simulink model "DARM"  (Simulink 7.5)
settings: Solver=ode45  StartTime=0.0  StopTime=10.0  RelTol=1e-3
values from neighbouring files (symbols this model uses):
  ifoParams = evalin('base', 'ifoParams')    [darmNbParams.m]
libraries: cstblocks x132, NbLibrary x29
(part 2 of 2)

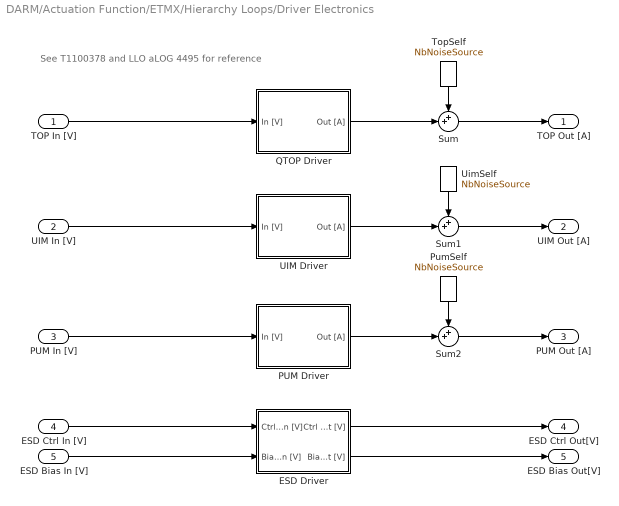
== system DARM/Actuation Function/ETMX/Hierarchy Loops/Driver Electronics ==
  note: See T1100378 and LLO aLOG 4495 for reference
  TOP In [V] : Inport
  UIM In [V] : Inport  Port=2
  PUM In [V] : Inport  Port=3
  ESD Ctrl In [V] : Inport  Port=4
  ESD Bias In [V] : Inport  Port=5
  ESD Driver : Subsystem
  PUM Driver : Subsystem  Description=FlexTf: ifoParams.act.drivers.pum.frd
      settings: AttributesFormatString=%<Description>
  PumSelf : NbLibrary/NbNoiseSource  Tag=NbNoiseSource  SystemSampleTime=-1  group='QUAD Actuator'  asd=ifoParams.darmNb.quadPumSelf
      settings: AttributesFormatString=%<Tag>
  QTOP Driver : Subsystem  Description=FlexTf: ifoParams.act.drivers.top.frd
      settings: AttributesFormatString=%<Description>
  Sum : Sum  Inputs=++|
  Sum1 : Sum  Inputs=++|
  Sum2 : Sum  Inputs=++|
  TopSelf : NbLibrary/NbNoiseSource  Tag=NbNoiseSource  SystemSampleTime=-1  group='QUAD Actuator'  asd=ifoParams.darmNb.quadTopSelf
      settings: AttributesFormatString=%<Tag>
  UIM Driver : Subsystem  Description=FlexTf: ifoParams.act.drivers.uim.frd
      settings: AttributesFormatString=%<Description>
  UimSelf : NbLibrary/NbNoiseSource  Tag=NbNoiseSource  SystemSampleTime=-1  group='QUAD Actuator'  asd=ifoParams.darmNb.quadUimSelf
      settings: AttributesFormatString=%<Tag>
  TOP Out [A] : Outport
  UIM Out [A] : Outport  Port=2
  PUM Out [A] : Outport  Port=3
  ESD Ctrl Out[V] : Outport  Port=4
  ESD Bias Out[V] : Outport  Port=5
  wires:
  TOP In [V]/1 -> QTOP Driver/1(In [V])
  PUM In [V]/1 -> PUM Driver/1(In [V])
  UIM In [V]/1 -> UIM Driver/1(In [V])
  ESD Driver/1(Ctrl Out [V]) -> ESD Ctrl Out[V]/1
  ESD Ctrl In [V]/1 -> ESD Driver/1(Ctrl In [V])
  ESD Driver/2(Bias Out [V]) -> ESD Bias Out[V]/1
  ESD Bias In [V]/1 -> ESD Driver/2(Bias In [V])
  TopSelf/1 -> Sum/1
  QTOP Driver/1(Out [A]) -> Sum/2
  Sum/1 -> TOP Out [A]/1
  UIM Driver/1(Out [A]) -> Sum1/2
  UimSelf/1 -> Sum1/1
  Sum1/1 -> UIM Out [A]/1
  PUM Driver/1(Out [A]) -> Sum2/2
  Sum2/1 -> PUM Out [A]/1
  PumSelf/1 -> Sum2/1

== system DARM/Actuation Function/ETMX/Hierarchy Loops/Driver Force Coefficient ==
  note: See T1100378
  note: Current to Force [N/A]
  note: Current to Force [N/A]
  note: Current to Force [N/A]
  In1[A] : Inport
  In2[A] : Inport  Port=2
  In3[A] : Inport  Port=3
  Vsig[V] : Inport  Port=4
  Vbias[V] : Inport  Port=5
  Gain : Gain  Gain=1.694
  Gain1 : Gain  Gain=1.694
  Gain2 : Gain  Gain=0.0309
  Gain7 : Gain  Gain=4.2e-10 / 4
  Math Function : Math  Operator=square  SaturateOnIntegerOverflow=on
  Subtract : Sum  Inputs=+-
  TOP_Out [N] : Outport
  UIM_Out [N] : Outport  Port=2
  PUM_Out [N] : Outport  Port=3
  TST_Out [N] : Outport  Port=4
  wires:
  In3[A]/1 -> Gain2/1
  In2[A]/1 -> Gain1/1
  In1[A]/1 -> Gain/1
  Gain2/1 -> PUM_Out [N]/1
  Gain1/1 -> UIM_Out [N]/1
  Gain/1 -> TOP_Out [N]/1
  Vsig[V]/1 -> Subtract/1
  Subtract/1 -> Math Function/1
  Math Function/1 -> Gain7/1
  Gain7/1 -> TST_Out [N]/1
  Vbias[V]/1 -> Subtract/2

== system DARM/Actuation Function/ETMX/Hierarchy Loops/EUL2OSEM ==
  note: 4 coil-magnet
      | actuators
  note: 4 coil-magnet
      | actuators
  note: 2 coil-magnet
      | actuators
  note: 4 ESD Quadrants
  M0_L_IN [ct] : Inport
  L1_L_IN [ct] : Inport  Port=2
  L2_L_IN [ct] : Inport  Port=3
  L3_L_IN [ct] : Inport  Port=4
  Gain1 : Gain  Gain=1/4
  Gain3 : Gain  Gain=1/2
  Gain4 : Gain  Gain=1/4
  Gain5 : Gain  Gain=1/4
  M0_OSEM_OUT [ct] : Outport
  L1_OSEM_OUT [ct] : Outport  Port=2
  L2_OSEM_OUT [ct] : Outport  Port=3
  L3_OSEM_OUT [ct] : Outport  Port=4
  wires:
  M0_L_IN [ct]/1 -> Gain3/1
  L1_L_IN [ct]/1 -> Gain4/1
  L2_L_IN [ct]/1 -> Gain5/1
  L3_L_IN [ct]/1 -> Gain1/1
  Gain3/1 -> M0_OSEM_OUT [ct]/1
  Gain4/1 -> L1_OSEM_OUT [ct]/1
  Gain5/1 -> L2_OSEM_OUT [ct]/1
  Gain1/1 -> L3_OSEM_OUT [ct]/1

== system DARM/Actuation Function/ETMX/Hierarchy Loops/L1 LOCK ==
  LSC_IN [m] : Inport
  FM1 : cstblocks/LTI System  Description=FlexTf: ifoParams.act.L1.lock(1).frd  SystemSampleTime=-1  sys=ifoParams.act.L1.lock(1).ss  IC=[]
      settings: AttributesFormatString=%<Description>
  FM10 : cstblocks/LTI System  SystemSampleTime=-1  sys=ifoParams.act.L1.lock(10).ss  IC=[]
  FM2 : cstblocks/LTI System  Description=FlexTf: ifoParams.act.L1.lock(2).frd  SystemSampleTime=-1  sys=ifoParams.act.L1.lock(2).ss  IC=[]
      settings: AttributesFormatString=%<Description>
  FM3 : cstblocks/LTI System  SystemSampleTime=-1  sys=ifoParams.act.L1.lock(3).ss  IC=[]
  FM4 : cstblocks/LTI System  SystemSampleTime=-1  sys=ifoParams.act.L1.lock(4).ss  IC=[]
  FM5 : cstblocks/LTI System  SystemSampleTime=-1  sys=ifoParams.act.L1.lock(5).ss  IC=[]
  FM6 : cstblocks/LTI System  SystemSampleTime=-1  sys=ifoParams.act.L1.lock(6).ss  IC=[]
  FM7 : cstblocks/LTI System  SystemSampleTime=-1  sys=ifoParams.act.L1.lock(7).ss  IC=[]
  FM8 : cstblocks/LTI System  SystemSampleTime=-1  sys=ifoParams.act.L1.lock(8).ss  IC=[]
  FM9 : cstblocks/LTI System  SystemSampleTime=-1  sys=ifoParams.act.L1.lock(9).ss  IC=[]
  Gain2 : Gain  Gain=ifoParams.act.L1.lockGain
  L1_OUT [ct] : Outport
  wires:
  FM1/1 -> FM2/1
  FM2/1 -> FM3/1
  FM3/1 -> FM4/1
  FM4/1 -> FM5/1
  FM6/1 -> FM7/1
  FM7/1 -> FM8/1
  FM8/1 -> FM9/1
  FM9/1 -> FM10/1
  LSC_IN [m]/1 -> FM1/1
  FM10/1 -> Gain2/1
  Gain2/1 -> L1_OUT [ct]/1
  FM5/1 -> FM6/1

== system DARM/Actuation Function/ETMX/Hierarchy Loops/L2 LOCK ==
  LSC_IN [m] : Inport
  FM1 : cstblocks/LTI System  Description=FlexTf: ifoParams.act.L2.lock(1).frd  SystemSampleTime=-1  sys=ifoParams.act.L2.lock(1).ss  IC=[]
      settings: AttributesFormatString=%<Description>
  FM10 : cstblocks/LTI System  SystemSampleTime=-1  sys=ifoParams.act.L2.lock(10).ss  IC=[]
  FM2 : cstblocks/LTI System  Description=FlexTf: ifoParams.act.L2.lock(2).frd  SystemSampleTime=-1  sys=ifoParams.act.L2.lock(2).ss  IC=[]
      settings: AttributesFormatString=%<Description>
  FM3 : cstblocks/LTI System  Description=FlexTf: ifoParams.act.L2.lock(3).frd  SystemSampleTime=-1  sys=ifoParams.act.L2.lock(3).ss  IC=[]
      settings: AttributesFormatString=%<Description>
  FM4 : cstblocks/LTI System  SystemSampleTime=-1  sys=ifoParams.act.L2.lock(4).ss  IC=[]
  FM5 : cstblocks/LTI System  SystemSampleTime=-1  sys=ifoParams.act.L2.lock(5).ss  IC=[]
  FM6 : cstblocks/LTI System  SystemSampleTime=-1  sys=ifoParams.act.L2.lock(6).ss  IC=[]
  FM7 : cstblocks/LTI System  SystemSampleTime=-1  sys=ifoParams.act.L2.lock(7).ss  IC=[]
  FM8 : cstblocks/LTI System  SystemSampleTime=-1  sys=ifoParams.act.L2.lock(8).ss  IC=[]
  FM9 : cstblocks/LTI System  SystemSampleTime=-1  sys=ifoParams.act.L2.lock(9).ss  IC=[]
  Gain2 : Gain  Gain=ifoParams.act.L2.lockGain
  L2_OUT [ct] : Outport
  wires:
  FM1/1 -> FM2/1
  FM2/1 -> FM3/1
  FM3/1 -> FM4/1
  FM4/1 -> FM5/1
  FM6/1 -> FM7/1
  FM7/1 -> FM8/1
  FM8/1 -> FM9/1
  FM9/1 -> FM10/1
  LSC_IN [m]/1 -> FM1/1
  FM10/1 -> Gain2/1
  Gain2/1 -> L2_OUT [ct]/1
  FM5/1 -> FM6/1

== system DARM/Actuation Function/ETMX/Hierarchy Loops/L3 LOCK ==
  LSC_IN [m] : Inport
  FM1 : cstblocks/LTI System  Description=FlexTf: ifoParams.act.L3.lock(1).frd  SystemSampleTime=-1  sys=ifoParams.act.L3.lock(1).ss  IC=[]
      settings: AttributesFormatString=%<Description>
  FM10 : cstblocks/LTI System  SystemSampleTime=-1  sys=ifoParams.act.L3.lock(10).ss  IC=[]
  FM2 : cstblocks/LTI System  Description=FlexTf: ifoParams.act.L3.lock(2).frd  SystemSampleTime=-1  sys=ifoParams.act.L3.lock(2).ss  IC=[]
      settings: AttributesFormatString=%<Description>
  FM3 : cstblocks/LTI System  Description=FlexTf: ifoParams.act.L3.lock(3).frd  SystemSampleTime=-1  sys=ifoParams.act.L3.lock(3).ss  IC=[]
      settings: AttributesFormatString=%<Description>
  FM4 : cstblocks/LTI System  SystemSampleTime=-1  sys=ifoParams.act.L3.lock(4).ss  IC=[]
  FM5 : cstblocks/LTI System  SystemSampleTime=-1  sys=ifoParams.act.L3.lock(5).ss  IC=[]
  FM6 : cstblocks/LTI System  SystemSampleTime=-1  sys=ifoParams.act.L3.lock(6).ss  IC=[]
  FM7 : cstblocks/LTI System  SystemSampleTime=-1  sys=ifoParams.act.L3.lock(7).ss  IC=[]
  FM8 : cstblocks/LTI System  SystemSampleTime=-1  sys=ifoParams.act.L3.lock(8).ss  IC=[]
  FM9 : cstblocks/LTI System  SystemSampleTime=-1  sys=ifoParams.act.L3.lock(9).ss  IC=[]
  Gain2 : Gain  Gain=ifoParams.act.L3.lockGain
  L3_OUT [ct] : Outport
  wires:
  FM1/1 -> FM2/1
  FM2/1 -> FM3/1
  FM3/1 -> FM4/1
  FM4/1 -> FM5/1
  FM6/1 -> FM7/1
  FM7/1 -> FM8/1
  FM8/1 -> FM9/1
  FM9/1 -> FM10/1
  LSC_IN [m]/1 -> FM1/1
  FM10/1 -> Gain2/1
  Gain2/1 -> L3_OUT [ct]/1
  FM5/1 -> FM6/1

== system DARM/Actuation Function/ETMX/Hierarchy Loops/LSC_ETMX ==
  LSC_ETMX_IN : Inport
  FM1 : cstblocks/LTI System  SystemSampleTime=-1  sys=ifoParams.act.lsc.etmx(1).ss  IC=[]
  FM10 : cstblocks/LTI System  SystemSampleTime=-1  sys=ifoParams.act.lsc.etmx(10).ss  IC=[]
  FM2 : cstblocks/LTI System  SystemSampleTime=-1  sys=ifoParams.act.lsc.etmx(2).ss  IC=[]
  FM3 : cstblocks/LTI System  SystemSampleTime=-1  sys=ifoParams.act.lsc.etmx(3).ss  IC=[]
  FM4 : cstblocks/LTI System  SystemSampleTime=-1  sys=ifoParams.act.lsc.etmx(4).ss  IC=[]
  FM5 : cstblocks/LTI System  SystemSampleTime=-1  sys=ifoParams.act.lsc.etmx(5).ss  IC=[]
  FM6 : cstblocks/LTI System  SystemSampleTime=-1  sys=ifoParams.act.lsc.etmx(6).ss  IC=[]
  FM7 : cstblocks/LTI System  SystemSampleTime=-1  sys=ifoParams.act.lsc.etmx(7).ss  IC=[]
  FM8 : cstblocks/LTI System  SystemSampleTime=-1  sys=ifoParams.act.lsc.etmx(8).ss  IC=[]
  FM9 : cstblocks/LTI System  SystemSampleTime=-1  sys=ifoParams.act.lsc.etmx(9).ss  IC=[]
  Gain2 : Gain  Gain=ifoParams.act.lsc.etmxGain
  "LSC_ETMX_OUT " : Outport
  wires:
  FM1/1 -> FM2/1
  FM2/1 -> FM3/1
  FM3/1 -> FM4/1
  FM4/1 -> FM5/1
  FM6/1 -> FM7/1
  FM7/1 -> FM8/1
  FM8/1 -> FM9/1
  FM9/1 -> FM10/1
  LSC_ETMX_IN/1 -> FM1/1
  FM10/1 -> Gain2/1
  Gain2/1 -> "LSC_ETMX_OUT "/1
  FM5/1 -> FM6/1

== system DARM/Actuation Function/ETMX/Hierarchy Loops/M0 LOCK ==
  LSC_IN [m] : Inport
  FM1 : cstblocks/LTI System  SystemSampleTime=-1  sys=ifoParams.act.M0.lock(1).ss  IC=[]
  FM10 : cstblocks/LTI System  SystemSampleTime=-1  sys=ifoParams.act.M0.lock(10).ss  IC=[]
  FM2 : cstblocks/LTI System  SystemSampleTime=-1  sys=ifoParams.act.M0.lock(2).ss  IC=[]
  FM3 : cstblocks/LTI System  SystemSampleTime=-1  sys=ifoParams.act.M0.lock(3).ss  IC=[]
  FM4 : cstblocks/LTI System  SystemSampleTime=-1  sys=ifoParams.act.M0.lock(4).ss  IC=[]
  FM5 : cstblocks/LTI System  SystemSampleTime=-1  sys=ifoParams.act.M0.lock(5).ss  IC=[]
  FM6 : cstblocks/LTI System  SystemSampleTime=-1  sys=ifoParams.act.M0.lock(6).ss  IC=[]
  FM7 : cstblocks/LTI System  SystemSampleTime=-1  sys=ifoParams.act.M0.lock(7).ss  IC=[]
  FM8 : cstblocks/LTI System  SystemSampleTime=-1  sys=ifoParams.act.M0.lock(8).ss  IC=[]
  FM9 : cstblocks/LTI System  SystemSampleTime=-1  sys=ifoParams.act.M0.lock(9).ss  IC=[]
  Gain2 : Gain  Gain=ifoParams.act.M0.lockGain
  M0_OUT [ct] : Outport
  wires:
  FM1/1 -> FM2/1
  FM2/1 -> FM3/1
  FM3/1 -> FM4/1
  FM4/1 -> FM5/1
  FM6/1 -> FM7/1
  FM7/1 -> FM8/1
  FM8/1 -> FM9/1
  FM9/1 -> FM10/1
  LSC_IN [m]/1 -> FM1/1
  FM10/1 -> Gain2/1
  Gain2/1 -> M0_OUT [ct]/1
  FM5/1 -> FM6/1

== system DARM/Actuation Function/ETMY/Hierarchy Loops/Actuator-to-Euler Transform ==
  note: 4 coil-magnet
      | actuators
  note: 4 coil-magnet
      | actuators
  note: 2 coil-magnet
      | actuators
  note: 4 ESD Quadrants
  TOP_OSEM_IN [N] : Inport
  UIM_OSEM_IN [N] : Inport  Port=2
  PUM_OSEM_IN [N] : Inport  Port=3
  TST_OSEM_IN [N] : Inport  Port=4
  Gain1 : Gain  Gain=4
  Gain3 : Gain  Gain=2
  Gain4 : Gain  Gain=4
  Gain5 : Gain  Gain=4
  TOP_L_OUT [N] : Outport
  UIM_L_OUT [N] : Outport  Port=2
  PUM_L_OUT [N] : Outport  Port=3
  TST_L_OUT [N] : Outport  Port=4
  wires:
  TOP_OSEM_IN [N]/1 -> Gain3/1
  Gain3/1 -> TOP_L_OUT [N]/1
  UIM_OSEM_IN [N]/1 -> Gain4/1
  Gain4/1 -> UIM_L_OUT [N]/1
  PUM_OSEM_IN [N]/1 -> Gain5/1
  Gain5/1 -> PUM_L_OUT [N]/1
  TST_OSEM_IN [N]/1 -> Gain1/1
  Gain1/1 -> TST_L_OUT [N]/1

== system DARM/Actuation Function/ETMY/Hierarchy Loops/Anti-Aliasing Chassis ==
  TOP In [V[ : Inport
  UIM In [V] : Inport  Port=2
  PUM In [V] : Inport  Port=3
  ESD Ctrl In [V] : Inport  Port=4
  ESD Bias In [V] : Inport  Port=5
  Gain{,1..4} (5 alike) : Gain
  TOP Out [V] : Outport
  UIM Out [V] : Outport  Port=2
  PUM Out[V] : Outport  Port=3
  ESD Ctrl Out V] : Outport  Port=4
  ESD Bias Out [V] : Outport  Port=5
  wires:
  Gain1/1 -> UIM Out [V]/1
  UIM In [V]/1 -> Gain1/1
  Gain2/1 -> PUM Out[V]/1
  PUM In [V]/1 -> Gain2/1
  Gain/1 -> TOP Out [V]/1
  TOP In [V[/1 -> Gain/1
  Gain3/1 -> ESD Ctrl Out V]/1
  ESD Ctrl In [V]/1 -> Gain3/1
  Gain4/1 -> ESD Bias Out [V]/1
  ESD Bias In [V]/1 -> Gain4/1

== system DARM/Actuation Function/ETMY/Hierarchy Loops/COILOUTF ==
  note: See T1100378 and LLO aLOG 4495 for reference
  M0_IN [ct] : Inport
  L1_IN [ct] : Inport  Port=2
  L2_IN [ct] : Inport  Port=3
  L3_CTRL_IN [ct] : Inport  Port=4
  L3_BIAS_IN [ct] : Inport  Port=5
  L1 : Subsystem
  L2 : Subsystem
  L3 : Subsystem
  M0 : Subsystem
  M0_OUT [ct] : Outport
  L1_OUT [ct] : Outport  Port=2
  L2_OUT [ct] : Outport  Port=3
  L3_CTRL_OUT [ct] : Outport  Port=4
  L3_BIAS_OUT [ct] : Outport  Port=5
  wires:
  M0/1(Out [ct]) -> M0_OUT [ct]/1
  M0_IN [ct]/1 -> M0/1(In [ct])
  L2_IN [ct]/1 -> L2/1(In [ct])
  L1_IN [ct]/1 -> L1/1(In [ct])
  L3/1(Ctrl Out [V]) -> L3_CTRL_OUT [ct]/1
  L3_CTRL_IN [ct]/1 -> L3/1(Ctrl In [V])
  L1/1(Out [ct]) -> L1_OUT [ct]/1
  L2/1(Out [ct]) -> L2_OUT [ct]/1
  L3/2(Bias Out [V]) -> L3_BIAS_OUT [ct]/1
  L3_BIAS_IN [ct]/1 -> L3/2(Bias In [V])

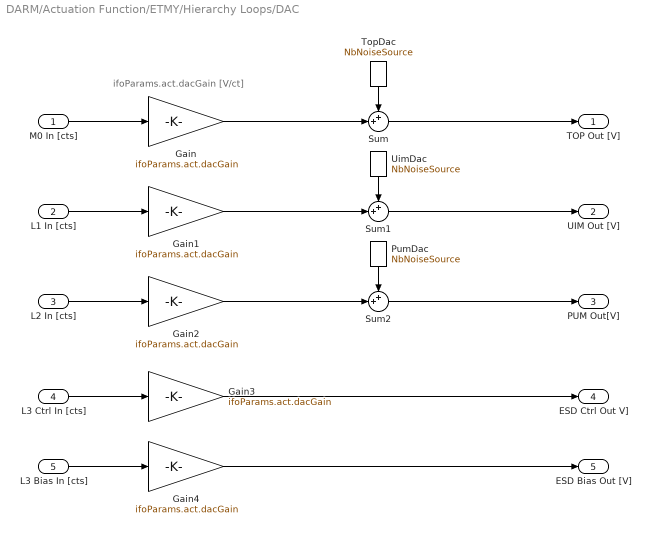
== system DARM/Actuation Function/ETMY/Hierarchy Loops/DAC ==
  note: ifoParams.act.dacGain
      | [V/ct]
  M0 In [cts] : Inport
  L1 In [cts] : Inport  Port=2
  L2 In [cts] : Inport  Port=3
  L3 Ctrl In [cts] : Inport  Port=4
  L3 Bias In [cts] : Inport  Port=5
  Gain{,1..4} (5 alike) : Gain  Gain=ifoParams.act.dacGain
  PumDac : NbLibrary/NbNoiseSource  Tag=NbNoiseSource  SystemSampleTime=-1  group='QUAD Actuator'  asd=ifoParams.darmNb.quadPumDac
      settings: AttributesFormatString=%<Tag>
  Sum : Sum  Inputs=++|
  Sum1 : Sum  Inputs=++|
  Sum2 : Sum  Inputs=++|
  TopDac : NbLibrary/NbNoiseSource  Tag=NbNoiseSource  SystemSampleTime=-1  group='QUAD Actuator'  asd=ifoParams.darmNb.quadTopDac
      settings: AttributesFormatString=%<Tag>
  UimDac : NbLibrary/NbNoiseSource  Tag=NbNoiseSource  SystemSampleTime=-1  group='QUAD Actuator'  asd=ifoParams.darmNb.quadUimDac
      settings: AttributesFormatString=%<Tag>
  TOP Out [V] : Outport
  UIM Out [V] : Outport  Port=2
  PUM Out[V] : Outport  Port=3
  ESD Ctrl Out V] : Outport  Port=4
  ESD Bias Out [V] : Outport  Port=5
  wires:
  L1 In [cts]/1 -> Gain1/1
  L2 In [cts]/1 -> Gain2/1
  M0 In [cts]/1 -> Gain/1
  L3 Ctrl In [cts]/1 -> Gain3/1
  Gain4/1 -> ESD Bias Out [V]/1
  L3 Bias In [cts]/1 -> Gain4/1
  Gain/1 -> Sum/2
  Sum/1 -> TOP Out [V]/1
  TopDac/1 -> Sum/1
  UimDac/1 -> Sum1/1
  Gain1/1 -> Sum1/2
  Sum1/1 -> UIM Out [V]/1
  Gain2/1 -> Sum2/2
  Sum2/1 -> PUM Out[V]/1
  PumDac/1 -> Sum2/1
  Gain3/1 -> ESD Ctrl Out V]/1

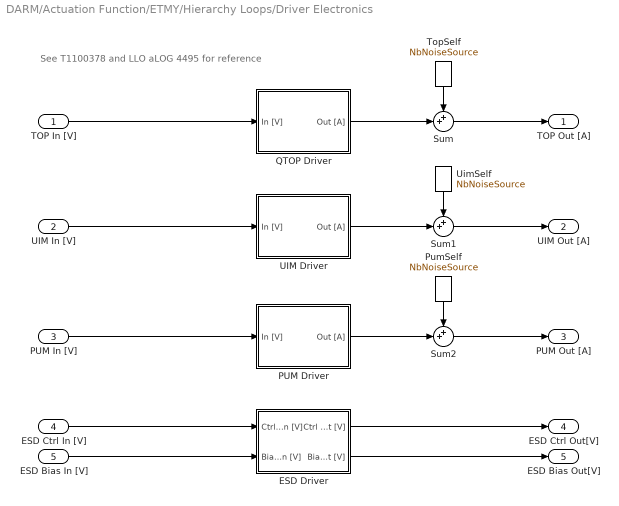
== system DARM/Actuation Function/ETMY/Hierarchy Loops/Driver Electronics ==
  note: See T1100378 and LLO aLOG 4495 for reference
  TOP In [V] : Inport
  UIM In [V] : Inport  Port=2
  PUM In [V] : Inport  Port=3
  ESD Ctrl In [V] : Inport  Port=4
  ESD Bias In [V] : Inport  Port=5
  ESD Driver : Subsystem
  PUM Driver : Subsystem  Description=FlexTf: ifoParams.act.drivers.pum.frd
      settings: AttributesFormatString=%<Description>
  PumSelf : NbLibrary/NbNoiseSource  Tag=NbNoiseSource  SystemSampleTime=-1  group='QUAD Actuator'  asd=ifoParams.darmNb.quadPumSelf
      settings: AttributesFormatString=%<Tag>
  QTOP Driver : Subsystem  Description=FlexTf: ifoParams.act.drivers.top.frd
      settings: AttributesFormatString=%<Description>
  Sum : Sum  Inputs=++|
  Sum1 : Sum  Inputs=++|
  Sum2 : Sum  Inputs=++|
  TopSelf : NbLibrary/NbNoiseSource  Tag=NbNoiseSource  SystemSampleTime=-1  group='QUAD Actuator'  asd=ifoParams.darmNb.quadTopSelf
      settings: AttributesFormatString=%<Tag>
  UIM Driver : Subsystem  Description=FlexTf: ifoParams.act.drivers.uim.frd
      settings: AttributesFormatString=%<Description>
  UimSelf : NbLibrary/NbNoiseSource  Tag=NbNoiseSource  SystemSampleTime=-1  group='QUAD Actuator'  asd=ifoParams.darmNb.quadUimSelf
      settings: AttributesFormatString=%<Tag>
  TOP Out [A] : Outport
  UIM Out [A] : Outport  Port=2
  PUM Out [A] : Outport  Port=3
  ESD Ctrl Out[V] : Outport  Port=4
  ESD Bias Out[V] : Outport  Port=5
  wires:
  TOP In [V]/1 -> QTOP Driver/1(In [V])
  PUM In [V]/1 -> PUM Driver/1(In [V])
  UIM In [V]/1 -> UIM Driver/1(In [V])
  ESD Driver/1(Ctrl Out [V]) -> ESD Ctrl Out[V]/1
  ESD Ctrl In [V]/1 -> ESD Driver/1(Ctrl In [V])
  ESD Driver/2(Bias Out [V]) -> ESD Bias Out[V]/1
  ESD Bias In [V]/1 -> ESD Driver/2(Bias In [V])
  QTOP Driver/1(Out [A]) -> Sum/2
  TopSelf/1 -> Sum/1
  Sum/1 -> TOP Out [A]/1
  UIM Driver/1(Out [A]) -> Sum1/2
  Sum1/1 -> UIM Out [A]/1
  UimSelf/1 -> Sum1/1
  PUM Driver/1(Out [A]) -> Sum2/2
  Sum2/1 -> PUM Out [A]/1
  PumSelf/1 -> Sum2/1

== system DARM/Actuation Function/ETMY/Hierarchy Loops/Driver Force Coefficient ==
  note: See T1100378
  note: Current to Force [N/A]
  note: Current to Force [N/A]
  note: Current to Force [N/A]
  In1[A] : Inport
  In2[A] : Inport  Port=2
  In3[A] : Inport  Port=3
  Vsig[V] : Inport  Port=4
  Vbias[V] : Inport  Port=5
  Gain : Gain  Gain=1.694
  Gain1 : Gain  Gain=1.694
  Gain2 : Gain  Gain=0.0309
  Gain7 : Gain  Gain=4.2e-10 / 4
  Math Function : Math  Operator=square  SaturateOnIntegerOverflow=on
  Subtract : Sum  Inputs=+-
  TOP_Out [N] : Outport
  UIM_Out [N] : Outport  Port=2
  PUM_Out [N] : Outport  Port=3
  TST_Out [N] : Outport  Port=4
  wires:
  In3[A]/1 -> Gain2/1
  In2[A]/1 -> Gain1/1
  In1[A]/1 -> Gain/1
  Gain2/1 -> PUM_Out [N]/1
  Gain1/1 -> UIM_Out [N]/1
  Gain/1 -> TOP_Out [N]/1
  Vsig[V]/1 -> Subtract/1
  Subtract/1 -> Math Function/1
  Math Function/1 -> Gain7/1
  Gain7/1 -> TST_Out [N]/1
  Vbias[V]/1 -> Subtract/2

== system DARM/Actuation Function/ETMY/Hierarchy Loops/EUL2OSEM ==
  note: 4 coil-magnet
      | actuators
  note: 4 coil-magnet
      | actuators
  note: 2 coil-magnet
      | actuators
  note: 4 ESD Quadrants
  M0_L_IN [ct] : Inport
  L1_L_IN [ct] : Inport  Port=2
  L2_L_IN [ct] : Inport  Port=3
  L3_L_IN [ct] : Inport  Port=4
  Gain1 : Gain  Gain=1/4
  Gain3 : Gain  Gain=1/2
  Gain4 : Gain  Gain=1/4
  Gain5 : Gain  Gain=1/4
  M0_OSEM_OUT [ct] : Outport
  L1_OSEM_OUT [ct] : Outport  Port=2
  L2_OSEM_OUT [ct] : Outport  Port=3
  L3_OSEM_OUT [ct] : Outport  Port=4
  wires:
  M0_L_IN [ct]/1 -> Gain3/1
  L1_L_IN [ct]/1 -> Gain4/1
  L2_L_IN [ct]/1 -> Gain5/1
  L3_L_IN [ct]/1 -> Gain1/1
  Gain3/1 -> M0_OSEM_OUT [ct]/1
  Gain4/1 -> L1_OSEM_OUT [ct]/1
  Gain5/1 -> L2_OSEM_OUT [ct]/1
  Gain1/1 -> L3_OSEM_OUT [ct]/1

== system DARM/Actuation Function/ETMY/Hierarchy Loops/L1 LOCK ==
  LSC_IN [m] : Inport
  FM1 : cstblocks/LTI System  Description=FlexTf: ifoParams.act.L1.lock(1).frd  SystemSampleTime=-1  sys=ifoParams.act.L1.lock(1).ss  IC=[]
      settings: AttributesFormatString=%<Description>
  FM10 : cstblocks/LTI System  SystemSampleTime=-1  sys=ifoParams.act.L1.lock(10).ss  IC=[]
  FM2 : cstblocks/LTI System  Description=FlexTf: ifoParams.act.L1.lock(2).frd  SystemSampleTime=-1  sys=ifoParams.act.L1.lock(2).ss  IC=[]
      settings: AttributesFormatString=%<Description>
  FM3 : cstblocks/LTI System  SystemSampleTime=-1  sys=ifoParams.act.L1.lock(3).ss  IC=[]
  FM4 : cstblocks/LTI System  SystemSampleTime=-1  sys=ifoParams.act.L1.lock(4).ss  IC=[]
  FM5 : cstblocks/LTI System  SystemSampleTime=-1  sys=ifoParams.act.L1.lock(5).ss  IC=[]
  FM6 : cstblocks/LTI System  SystemSampleTime=-1  sys=ifoParams.act.L1.lock(6).ss  IC=[]
  FM7 : cstblocks/LTI System  SystemSampleTime=-1  sys=ifoParams.act.L1.lock(7).ss  IC=[]
  FM8 : cstblocks/LTI System  SystemSampleTime=-1  sys=ifoParams.act.L1.lock(8).ss  IC=[]
  FM9 : cstblocks/LTI System  SystemSampleTime=-1  sys=ifoParams.act.L1.lock(9).ss  IC=[]
  Gain2 : Gain  Gain=ifoParams.act.L1.lockGain
  L1_OUT [ct] : Outport
  wires:
  FM1/1 -> FM2/1
  FM2/1 -> FM3/1
  FM3/1 -> FM4/1
  FM4/1 -> FM5/1
  FM6/1 -> FM7/1
  FM7/1 -> FM8/1
  FM8/1 -> FM9/1
  FM9/1 -> FM10/1
  LSC_IN [m]/1 -> FM1/1
  FM10/1 -> Gain2/1
  Gain2/1 -> L1_OUT [ct]/1
  FM5/1 -> FM6/1

== system DARM/Actuation Function/ETMY/Hierarchy Loops/L2 LOCK ==
  LSC_IN [m] : Inport
  FM1 : cstblocks/LTI System  Description=FlexTf: ifoParams.act.L2.lock(1).frd  SystemSampleTime=-1  sys=ifoParams.act.L2.lock(1).ss  IC=[]
      settings: AttributesFormatString=%<Description>
  FM10 : cstblocks/LTI System  SystemSampleTime=-1  sys=ifoParams.act.L2.lock(10).ss  IC=[]
  FM2 : cstblocks/LTI System  Description=FlexTf: ifoParams.act.L2.lock(2).frd  SystemSampleTime=-1  sys=ifoParams.act.L2.lock(2).ss  IC=[]
      settings: AttributesFormatString=%<Description>
  FM3 : cstblocks/LTI System  Description=FlexTf: ifoParams.act.L2.lock(3).frd  SystemSampleTime=-1  sys=ifoParams.act.L2.lock(3).ss  IC=[]
      settings: AttributesFormatString=%<Description>
  FM4 : cstblocks/LTI System  SystemSampleTime=-1  sys=ifoParams.act.L2.lock(4).ss  IC=[]
  FM5 : cstblocks/LTI System  SystemSampleTime=-1  sys=ifoParams.act.L2.lock(5).ss  IC=[]
  FM6 : cstblocks/LTI System  SystemSampleTime=-1  sys=ifoParams.act.L2.lock(6).ss  IC=[]
  FM7 : cstblocks/LTI System  SystemSampleTime=-1  sys=ifoParams.act.L2.lock(7).ss  IC=[]
  FM8 : cstblocks/LTI System  SystemSampleTime=-1  sys=ifoParams.act.L2.lock(8).ss  IC=[]
  FM9 : cstblocks/LTI System  SystemSampleTime=-1  sys=ifoParams.act.L2.lock(9).ss  IC=[]
  Gain2 : Gain  Gain=ifoParams.act.L2.lockGain
  L2_OUT [ct] : Outport
  wires:
  FM1/1 -> FM2/1
  FM2/1 -> FM3/1
  FM3/1 -> FM4/1
  FM4/1 -> FM5/1
  FM6/1 -> FM7/1
  FM7/1 -> FM8/1
  FM8/1 -> FM9/1
  FM9/1 -> FM10/1
  LSC_IN [m]/1 -> FM1/1
  FM10/1 -> Gain2/1
  Gain2/1 -> L2_OUT [ct]/1
  FM5/1 -> FM6/1

== system DARM/Actuation Function/ETMY/Hierarchy Loops/L3 LOCK ==
  LSC_IN [m] : Inport
  FM1 : cstblocks/LTI System  Description=FlexTf: ifoParams.act.L3.lock(1).frd  SystemSampleTime=-1  sys=ifoParams.act.L3.lock(1).ss  IC=[]
      settings: AttributesFormatString=%<Description>
  FM10 : cstblocks/LTI System  SystemSampleTime=-1  sys=ifoParams.act.L3.lock(10).ss  IC=[]
  FM2 : cstblocks/LTI System  Description=FlexTf: ifoParams.act.L3.lock(2).frd  SystemSampleTime=-1  sys=ifoParams.act.L3.lock(2).ss  IC=[]
      settings: AttributesFormatString=%<Description>
  FM3 : cstblocks/LTI System  Description=FlexTf: ifoParams.act.L3.lock(3).frd  SystemSampleTime=-1  sys=ifoParams.act.L3.lock(3).ss  IC=[]
      settings: AttributesFormatString=%<Description>
  FM4 : cstblocks/LTI System  SystemSampleTime=-1  sys=ifoParams.act.L3.lock(4).ss  IC=[]
  FM5 : cstblocks/LTI System  SystemSampleTime=-1  sys=ifoParams.act.L3.lock(5).ss  IC=[]
  FM6 : cstblocks/LTI System  SystemSampleTime=-1  sys=ifoParams.act.L3.lock(6).ss  IC=[]
  FM7 : cstblocks/LTI System  SystemSampleTime=-1  sys=ifoParams.act.L3.lock(7).ss  IC=[]
  FM8 : cstblocks/LTI System  SystemSampleTime=-1  sys=ifoParams.act.L3.lock(8).ss  IC=[]
  FM9 : cstblocks/LTI System  SystemSampleTime=-1  sys=ifoParams.act.L3.lock(9).ss  IC=[]
  Gain2 : Gain  Gain=ifoParams.act.L3.lockGain
  L3_OUT [ct] : Outport
  wires:
  FM1/1 -> FM2/1
  FM2/1 -> FM3/1
  FM3/1 -> FM4/1
  FM4/1 -> FM5/1
  FM6/1 -> FM7/1
  FM7/1 -> FM8/1
  FM8/1 -> FM9/1
  FM9/1 -> FM10/1
  LSC_IN [m]/1 -> FM1/1
  FM10/1 -> Gain2/1
  Gain2/1 -> L3_OUT [ct]/1
  FM5/1 -> FM6/1

== system DARM/Actuation Function/ETMY/Hierarchy Loops/LSC_ETMY ==
  LSC_ETMX_IN : Inport
  FM1 : cstblocks/LTI System  SystemSampleTime=-1  sys=ifoParams.act.lsc.etmx(1).ss  IC=[]
  FM10 : cstblocks/LTI System  SystemSampleTime=-1  sys=ifoParams.act.lsc.etmx(10).ss  IC=[]
  FM2 : cstblocks/LTI System  SystemSampleTime=-1  sys=ifoParams.act.lsc.etmx(2).ss  IC=[]
  FM3 : cstblocks/LTI System  SystemSampleTime=-1  sys=ifoParams.act.lsc.etmx(3).ss  IC=[]
  FM4 : cstblocks/LTI System  SystemSampleTime=-1  sys=ifoParams.act.lsc.etmx(4).ss  IC=[]
  FM5 : cstblocks/LTI System  SystemSampleTime=-1  sys=ifoParams.act.lsc.etmx(5).ss  IC=[]
  FM6 : cstblocks/LTI System  SystemSampleTime=-1  sys=ifoParams.act.lsc.etmx(6).ss  IC=[]
  FM7 : cstblocks/LTI System  SystemSampleTime=-1  sys=ifoParams.act.lsc.etmx(7).ss  IC=[]
  FM8 : cstblocks/LTI System  SystemSampleTime=-1  sys=ifoParams.act.lsc.etmx(8).ss  IC=[]
  FM9 : cstblocks/LTI System  SystemSampleTime=-1  sys=ifoParams.act.lsc.etmx(9).ss  IC=[]
  Gain2 : Gain  Gain=ifoParams.act.lsc.etmxGain
  "LSC_ETMX_OUT " : Outport
  wires:
  FM1/1 -> FM2/1
  FM2/1 -> FM3/1
  FM3/1 -> FM4/1
  FM4/1 -> FM5/1
  FM6/1 -> FM7/1
  FM7/1 -> FM8/1
  FM8/1 -> FM9/1
  FM9/1 -> FM10/1
  LSC_ETMX_IN/1 -> FM1/1
  FM10/1 -> Gain2/1
  Gain2/1 -> "LSC_ETMX_OUT "/1
  FM5/1 -> FM6/1

== system DARM/Actuation Function/ETMY/Hierarchy Loops/M0 LOCK ==
  LSC_IN [m] : Inport
  FM1 : cstblocks/LTI System  SystemSampleTime=-1  sys=ifoParams.act.M0.lock(1).ss  IC=[]
  FM10 : cstblocks/LTI System  SystemSampleTime=-1  sys=ifoParams.act.M0.lock(10).ss  IC=[]
  FM2 : cstblocks/LTI System  SystemSampleTime=-1  sys=ifoParams.act.M0.lock(2).ss  IC=[]
  FM3 : cstblocks/LTI System  SystemSampleTime=-1  sys=ifoParams.act.M0.lock(3).ss  IC=[]
  FM4 : cstblocks/LTI System  SystemSampleTime=-1  sys=ifoParams.act.M0.lock(4).ss  IC=[]
  FM5 : cstblocks/LTI System  SystemSampleTime=-1  sys=ifoParams.act.M0.lock(5).ss  IC=[]
  FM6 : cstblocks/LTI System  SystemSampleTime=-1  sys=ifoParams.act.M0.lock(6).ss  IC=[]
  FM7 : cstblocks/LTI System  SystemSampleTime=-1  sys=ifoParams.act.M0.lock(7).ss  IC=[]
  FM8 : cstblocks/LTI System  SystemSampleTime=-1  sys=ifoParams.act.M0.lock(8).ss  IC=[]
  FM9 : cstblocks/LTI System  SystemSampleTime=-1  sys=ifoParams.act.M0.lock(9).ss  IC=[]
  Gain2 : Gain  Gain=ifoParams.act.M0.lockGain
  M0_OUT [ct] : Outport
  wires:
  FM1/1 -> FM2/1
  FM2/1 -> FM3/1
  FM3/1 -> FM4/1
  FM4/1 -> FM5/1
  FM6/1 -> FM7/1
  FM7/1 -> FM8/1
  FM8/1 -> FM9/1
  FM9/1 -> FM10/1
  LSC_IN [m]/1 -> FM1/1
  FM10/1 -> Gain2/1
  Gain2/1 -> M0_OUT [ct]/1
  FM5/1 -> FM6/1

== system DARM/Sensing Function/DCPD Analog Electronics/Preamps/Preamp_PD1 ==
  note: Switches pass upper path if set to 1 (one),
      | lower path if set to 0 (zero)
  note: Zeros and Poles Derived from Schematic
      | (with more precision than the frequencies noted above the stages)
      | D060572-v1 (or B3).
  In [A] : Inport
  DC Transimpedance De-energized : Gain  Gain=100
  DC Transimpedance Energized : Gain  Gain=400
  Switch : Switch  Threshold=0.5
  Whitening_1  [7.3:79] : ZeroPole  Zeros=-2*pi*[7.3]  Poles=-2*pi*[79]  Gain=[79/7.3]
  Whitening_2 [7.3:79] : ZeroPole  Zeros=-2*pi*[7.3]  Poles=-2*pi*[79]  Gain=[79/7.3]
  ifoParams.sens.preamp.zswitch.state : Constant  Value=ifoParams.sens.preamp.zswitch.state
  Out [V] : Outport
  wires:
  In [A]/1 -> DC Transimpedance Energized/1, DC Transimpedance De-energized/1
  Whitening_2 [7.3:79]/1 -> Out [V]/1
  DC Transimpedance Energized/1 -> Switch/1
  Whitening_1  [7.3:79]/1 -> Whitening_2 [7.3:79]/1
  ifoParams.sens.preamp.zswitch.state/1 -> Switch/2
  DC Transimpedance De-energized/1 -> Switch/3
  Switch/1 -> Whitening_1  [7.3:79]/1

== system DARM/Sensing Function/DCPD Analog Electronics/Preamps/Preamp_PD2 ==
  note: Switches pass upper path if set to 1 (one),
      | lower path if set to 0 (zero)
  note: Zeros and Poles Derived from Schematic
      | (with more precision than the frequencies noted above the stages)
      | D060572-v1 (or B3).
  In [A] : Inport
  DC Transimpedance De-energized : Gain  Gain=100
  DC Transimpedance Energized : Gain  Gain=400
  Switch : Switch  Threshold=0.5
  Whitening_1  [7.3:79] : ZeroPole  Zeros=-2*pi*[7.3]  Poles=-2*pi*[79]  Gain=[79/7.3]
  Whitening_2 [7.3:79] : ZeroPole  Zeros=-2*pi*[7.3]  Poles=-2*pi*[79]  Gain=[79/7.3]
  ifoParams.sens.preamp.zswitch.state : Constant  Value=ifoParams.sens.preamp.zswitch.state
  Out [V] : Outport
  wires:
  In [A]/1 -> DC Transimpedance Energized/1, DC Transimpedance De-energized/1
  Whitening_2 [7.3:79]/1 -> Out [V]/1
  DC Transimpedance Energized/1 -> Switch/1
  Whitening_1  [7.3:79]/1 -> Whitening_2 [7.3:79]/1
  ifoParams.sens.preamp.zswitch.state/1 -> Switch/2
  DC Transimpedance De-energized/1 -> Switch/3
  Switch/1 -> Whitening_1  [7.3:79]/1

== system DARM/Sensing Function/DCPD Analog Electronics/Whitening Chassis/Whitening_PD1 ==
  note: Switches pass upper path if set to 1 (one),
      | lower path if set to 0 (zero)
  note: Zeros and Poles Derived from Schematic
      | (with more precision than the frequencies noted above the stages)
      | D070281-v1
  In [V] : Inport
  DC Gain : Gain  Gain=0.5
  Switch : Switch  Threshold=0.5
  Switch1 : Switch  Threshold=0.5
  Whitening_1  [7.3:79] : ZeroPole  Zeros=-2*pi*[7.3]  Poles=-2*pi*[79]  Gain=[79/7.3]
  Whitening_2 [24:260] : ZeroPole  Zeros=-2*pi*[24]  Poles=-2*pi*[260]  Gain=[260/24]
  ifoParams.sens.whitening.stage1.state : Constant  Value=ifoParams.sens.whitening.stage1.state
  ifoParams.sens.whitening.stage2.state : Constant  Value=ifoParams.sens.whitening.stage2.state
  Out [V] : Outport
  wires:
  DC Gain/1 -> Switch/1, Whitening_1  [7.3:79]/1
  In [V]/1 -> DC Gain/1
  ifoParams.sens.whitening.stage1.state/1 -> Switch/2
  Whitening_1  [7.3:79]/1 -> Switch/3
  Whitening_2 [24:260]/1 -> Switch1/3
  Switch/1 -> Switch1/1, Whitening_2 [24:260]/1
  Switch1/1 -> Out [V]/1
  ifoParams.sens.whitening.stage2.state/1 -> Switch1/2

== system DARM/Sensing Function/DCPD Analog Electronics/Whitening Chassis/Whitening_PD2 ==
  note: Switches pass upper path if set to 1 (one),
      | lower path if set to 0 (zero)
  note: Zeros and Poles Derived from Schematic
      | (with more precision than the frequencies noted above the stages)
      | D070281-v1
  In [V] : Inport
  DC Gain : Gain  Gain=0.5
  Switch : Switch  Threshold=0.5
  Switch1 : Switch  Threshold=0.5
  Whitening_1  [7.3:79] : ZeroPole  Zeros=-2*pi*[7.3]  Poles=-2*pi*[79]  Gain=[79/7.3]
  Whitening_2 [24:260] : ZeroPole  Zeros=-2*pi*[24]  Poles=-2*pi*[260]  Gain=[260/24]
  ifoParams.sens.whitening.stage1.state : Constant  Value=ifoParams.sens.whitening.stage1.state
  ifoParams.sens.whitening.stage2.state : Constant  Value=ifoParams.sens.whitening.stage2.state
  Out [V] : Outport
  wires:
  DC Gain/1 -> Switch/1, Whitening_1  [7.3:79]/1
  In [V]/1 -> DC Gain/1
  ifoParams.sens.whitening.stage1.state/1 -> Switch/2
  Whitening_1  [7.3:79]/1 -> Switch/3
  Whitening_2 [24:260]/1 -> Switch1/3
  Switch/1 -> Switch1/1, Whitening_2 [24:260]/1
  Switch1/1 -> Out [V]/1
  ifoParams.sens.whitening.stage2.state/1 -> Switch1/2

== system DARM/Sensing Function/DCPD Signal Conditioning/ISCINF/AntiPreamps_PD1 ==
  In [ct] : Inport
  AntiWhitening_1  [7.3:79] : ZeroPole  Zeros=-2*pi*[79]  Poles=-2*pi*[7.3]  Gain=[7.3/79]
  AntiWhitening_2  [7.3:79] : ZeroPole  Zeros=-2*pi*[79]  Poles=-2*pi*[7.3]  Gain=[7.3/79]
  Out [ct] : Outport
  wires:
  AntiWhitening_1  [7.3:79]/1 -> AntiWhitening_2  [7.3:79]/1
  In [ct]/1 -> AntiWhitening_1  [7.3:79]/1
  AntiWhitening_2  [7.3:79]/1 -> Out [ct]/1

== system DARM/Sensing Function/DCPD Signal Conditioning/ISCINF/AntiPreamps_PD2 ==
  In [ct] : Inport
  AntiWhitening_1  [7.3:79] : ZeroPole  Zeros=-2*pi*[79]  Poles=-2*pi*[7.3]  Gain=[7.3/79]
  AntiWhitening_2  [7.3:79] : ZeroPole  Zeros=-2*pi*[79]  Poles=-2*pi*[7.3]  Gain=[7.3/79]
  Out [ct] : Outport
  wires:
  AntiWhitening_1  [7.3:79]/1 -> AntiWhitening_2  [7.3:79]/1
  In [ct]/1 -> AntiWhitening_1  [7.3:79]/1
  AntiWhitening_2  [7.3:79]/1 -> Out [ct]/1

== system DARM/Sensing Function/DCPD Signal Conditioning/ISCINF/AntiWhitening_PD1 ==
  note: Switches pass upper path if set to 1 (one),
      | lower path if set to 0 (zero)
  note: Zeros and Poles Derived from Schematic
      | (with more precision than the frequencies noted above the stages)
      | D070281-v1
  In [ct] : Inport
  AntiWhitening_1  [7.3:79] : ZeroPole  Zeros=-2*pi*[79]  Poles=-2*pi*[7.3]  Gain=[7.3/79]
  AntiWhitening_2 [24:260] : ZeroPole  Zeros=-2*pi*[260]  Poles=-2*pi*[24]  Gain=[24/260]
  Switch : Switch  Threshold=0.5
  Switch1 : Switch  Threshold=0.5
  ifoParams.sens.whitening.stage1.state : Constant  Value=ifoParams.sens.whitening.stage1.state
  ifoParams.sens.whitening.stage2.state : Constant  Value=ifoParams.sens.whitening.stage2.state
  Out [ct] : Outport
  wires:
  In [ct]/1 -> Switch/1, AntiWhitening_1  [7.3:79]/1
  ifoParams.sens.whitening.stage1.state/1 -> Switch/2
  AntiWhitening_1  [7.3:79]/1 -> Switch/3
  AntiWhitening_2 [24:260]/1 -> Switch1/3
  Switch/1 -> Switch1/1, AntiWhitening_2 [24:260]/1
  Switch1/1 -> Out [ct]/1
  ifoParams.sens.whitening.stage2.state/1 -> Switch1/2

== system DARM/Sensing Function/DCPD Signal Conditioning/ISCINF/AntiWhitening_PD2 ==
  note: Switches pass upper path if set to 1 (one),
      | lower path if set to 0 (zero)
  note: Zeros and Poles Derived from Schematic
      | (with more precision than the frequencies noted above the stages)
      | D070281-v1
  In [ct] : Inport
  AntiWhitening_1  [7.3:79] : ZeroPole  Zeros=-2*pi*[79]  Poles=-2*pi*[7.3]  Gain=[7.3/79]
  AntiWhitening_2 [24:260] : ZeroPole  Zeros=-2*pi*[260]  Poles=-2*pi*[24]  Gain=[24/260]
  Switch : Switch  Threshold=0.5
  Switch1 : Switch  Threshold=0.5
  ifoParams.sens.whitening.stage1.state : Constant  Value=ifoParams.sens.whitening.stage1.state
  ifoParams.sens.whitening.stage2.state : Constant  Value=ifoParams.sens.whitening.stage2.state
  Out [ct] : Outport
  wires:
  In [ct]/1 -> Switch/1, AntiWhitening_1  [7.3:79]/1
  ifoParams.sens.whitening.stage1.state/1 -> Switch/2
  AntiWhitening_1  [7.3:79]/1 -> Switch/3
  AntiWhitening_2 [24:260]/1 -> Switch1/3
  Switch/1 -> Switch1/1, AntiWhitening_2 [24:260]/1
  Switch1/1 -> Out [ct]/1
  ifoParams.sens.whitening.stage2.state/1 -> Switch1/2

== system DARM/Actuation Function/ETMX/Hierarchy Loops/COILOUTF/L1 ==
  note: Switches pass upper path if set to 1 (one),
      | lower path if set to 0 (zero)
  In [ct] : Inport
  Switch : Switch  Threshold=0.5
  Switch1 : Switch  Threshold=0.5
  Switch2 : Switch  Threshold=0.5
  antiAcq [10:1] : ZeroPole  Zeros=-2*pi*[300]  Poles=-2*pi*[50]  Gain=[50/300]
  antiLP1 [1:10.5] : ZeroPole  Zeros=-2*pi*[1]  Poles=-2*pi*[10.5]  Gain=[10.5/1]
  antiLP2 [1:10.5] : ZeroPole  Zeros=-2*pi*[1]  Poles=-2*pi*[10.5]  Gain=[10.5/1]
  antiLP3 [1:10.5] : ZeroPole  Zeros=-2*pi*[1]  Poles=-2*pi*[10.5]  Gain=[10.5/1]
  drivers.uim.state.lp1 : Constant  Value=ifoParams.act.drivers.uim.state.lp1
  drivers.uim.state.lp2 : Constant  Value=ifoParams.act.drivers.uim.state.lp2
  drivers.uim.state.lp3 : Constant  Value=ifoParams.act.drivers.uim.state.lp3
  Out [ct] : Outport
  wires:
  drivers.uim.state.lp1/1 -> Switch/2
  antiLP1 [1:10.5]/1 -> Switch/1
  Switch/1 -> Switch1/3, antiLP2 [1:10.5]/1
  antiLP2 [1:10.5]/1 -> Switch1/1
  drivers.uim.state.lp2/1 -> Switch1/2
  Switch1/1 -> Switch2/3, antiLP3 [1:10.5]/1
  antiLP3 [1:10.5]/1 -> Switch2/1
  drivers.uim.state.lp3/1 -> Switch2/2
  In [ct]/1 -> antiLP1 [1:10.5]/1, Switch/3
  Switch2/1 -> antiAcq [10:1]/1
  antiAcq [10:1]/1 -> Out [ct]/1

== system DARM/Actuation Function/ETMX/Hierarchy Loops/COILOUTF/L2 ==
  note: Switches pass upper path if set to 1 (one),
      | lower path if set to 0 (zero)
  In [ct] : Inport
  Switch : Switch  Threshold=0.5
  Switch1 : Switch  Threshold=0.5
  antiAcqOff [110:12] : ZeroPole  Zeros=-2*pi*[110]  Poles=-2*pi*[12]  Gain=12/110
  antiAcqOn [80.5:1.35] : ZeroPole  Zeros=-2*pi*[80.5]  Poles=-2*pi*[1.35]  Gain=1.35/80.5
  antiLpOn [(0.5 250):(6 20)] : ZeroPole  Zeros=-2*pi*[0.5 250]  Poles=-2*pi*[6 20]  Gain=(6*20)/(0.5*250)
  drivers.pum.state.lp : Constant  Value=ifoParams.act.drivers.pum.state.lp
  drivers.top.state.acq : Constant  Value=ifoParams.act.drivers.pum.state.acq
  Out [ct] : Outport
  wires:
  drivers.pum.state.lp/1 -> Switch/2
  Switch/1 -> antiAcqOn [80.5:1.35]/1, antiAcqOff [110:12]/1
  antiAcqOn [80.5:1.35]/1 -> Switch1/1
  drivers.top.state.acq/1 -> Switch1/2
  In [ct]/1 -> antiLpOn [(0.5 250):(6 20)]/1, Switch/3
  Switch1/1 -> Out [ct]/1
  antiLpOn [(0.5 250):(6 20)]/1 -> Switch/1
  antiAcqOff [110:12]/1 -> Switch1/3

== system DARM/Actuation Function/ETMX/Hierarchy Loops/COILOUTF/L3 ==
  note: 2 kHz Pole is not digitally compensated
  Ctrl In [V] : Inport
  Bias In [V] : Inport  Port=2
  Ctrl Out [V] : Outport
  Bias Out [V] : Outport  Port=2
  wires:
  Ctrl In [V]/1 -> Ctrl Out [V]/1
  Bias In [V]/1 -> Bias Out [V]/1

== system DARM/Actuation Function/ETMX/Hierarchy Loops/COILOUTF/M0 ==
  note: Switches pass upper path if set to 1 (one),
      | lower path if set to 0 (zero)
  In [ct] : Inport
  Switch : Switch  Threshold=0.5
  antiAcq [1:31] : ZeroPole  Zeros=-2*pi*[1]  Poles=-2*pi*[31]  Gain=[31/1]
  antiLP [1:10] : ZeroPole  Zeros=-2*pi*[1]  Poles=-2*pi*[10]  Gain=[10/1]
  drivers.top.state.lp : Constant  Value=ifoParams.act.drivers.top.state.lp
  Out [ct] : Outport
  wires:
  Switch/1 -> antiAcq [1:31]/1
  antiLP [1:10]/1 -> Switch/1
  In [ct]/1 -> antiLP [1:10]/1, Switch/3
  antiAcq [1:31]/1 -> Out [ct]/1
  drivers.top.state.lp/1 -> Switch/2

== system DARM/Actuation Function/ETMX/Hierarchy Loops/Driver Electronics/ESD Driver ==
  Ctrl In [V] : Inport
  Bias In [V] : Inport  Port=2
  DC Gain1 : Gain  Gain=1.1
  DC Gain3 : Gain  Gain=1.1
  L3_ESD_filter [(none):(2000)] : ZeroPole  Zeros=[]  Poles=-2*pi*[2000]  Gain=[2*pi*2000]
  L3_ESD_filter [(none):(2000)]1 : ZeroPole  Zeros=[]  Poles=-2*pi*[2000]  Gain=[2*pi*2000]
  Ctrl Out [V] : Outport
  Bias Out [V] : Outport  Port=2
  wires:
  DC Gain3/1 -> L3_ESD_filter [(none):(2000)]/1
  Ctrl In [V]/1 -> DC Gain3/1
  L3_ESD_filter [(none):(2000)]/1 -> Ctrl Out [V]/1
  Bias In [V]/1 -> DC Gain1/1
  DC Gain1/1 -> L3_ESD_filter [(none):(2000)]1/1
  L3_ESD_filter [(none):(2000)]1/1 -> Bias Out [V]/1

== system DARM/Actuation Function/ETMX/Hierarchy Loops/Driver Electronics/PUM Driver ==
  note: Switches pass upper path if set to 1 (one),
      | lower path if set to 0 (zero)
  In [V] : Inport
  DC Transconductance : Gain  Gain=0.27e-3
  L2_ACQOFF_filter [12:110] : ZeroPole  Zeros=-2*pi*[12]  Poles=-2*pi*[110]  Gain=110/12
  L2_ACQON_filter [1.35:80.5] : ZeroPole  Zeros=-2*pi*[1.35]  Poles=-2*pi*[80.5]  Gain=80.5/1.35
  L2_LPON_filter [(0.5 250):(6 20)] : ZeroPole  Zeros=-2*pi*[6 20]  Poles=-2*pi*[0.5 250]  Gain=(0.5*250)/(6*20)
  Switch : Switch  Threshold=0.5
  Switch1 : Switch  Threshold=0.5
  drivers.pum.state.lp : Constant  Value=ifoParams.act.drivers.pum.state.lp
  drivers.top.state.acq : Constant  Value=ifoParams.act.drivers.pum.state.acq
  Out [A] : Outport
  wires:
  DC Transconductance/1 -> L2_LPON_filter [(0.5 250):(6 20)]/1, Switch/3
  drivers.pum.state.lp/1 -> Switch/2
  Switch/1 -> L2_ACQOFF_filter [12:110]/1, L2_ACQON_filter [1.35:80.5]/1
  L2_ACQON_filter [1.35:80.5]/1 -> Switch1/1
  drivers.top.state.acq/1 -> Switch1/2
  In [V]/1 -> DC Transconductance/1
  Switch1/1 -> Out [A]/1
  L2_LPON_filter [(0.5 250):(6 20)]/1 -> Switch/1
  L2_ACQOFF_filter [12:110]/1 -> Switch1/3

== system DARM/Actuation Function/ETMX/Hierarchy Loops/Driver Electronics/QTOP Driver ==
  note: Switches pass upper path if set to 1 (one),
      | lower path if set to 0 (zero)
  In [V] : Inport
  DC Transconductance : Gain  Gain=9.9e-3
  LP_filter [10:1] : ZeroPole  Zeros=-2*pi*[10]  Poles=-2*pi*[1]  Gain=[1/10]
  M0_Output_Filter [31:0.9] : ZeroPole  Zeros=-2*pi*[31]  Poles=-2*pi*[0.9]  Gain=[0.9/31]
  Switch : Switch  Threshold=0.5
  drivers.top.state.lp : Constant  Value=ifoParams.act.drivers.top.state.lp
  Out [A] : Outport
  wires:
  Switch/1 -> M0_Output_Filter [31:0.9]/1
  LP_filter [10:1]/1 -> Switch/1
  DC Transconductance/1 -> LP_filter [10:1]/1, Switch/3
  In [V]/1 -> DC Transconductance/1
  M0_Output_Filter [31:0.9]/1 -> Out [A]/1
  drivers.top.state.lp/1 -> Switch/2

== system DARM/Actuation Function/ETMX/Hierarchy Loops/Driver Electronics/UIM Driver ==
  note: Switches pass upper path if set to 1 (one),
      | lower path if set to 0 (zero)
  In [V] : Inport
  DC Transconductance : Gain  Gain=0.15e-3
  L1_LP1_filter [10.5:1] : ZeroPole  Zeros=-2*pi*[10.5]  Poles=-2*pi*[1]  Gain=[1/10.5]
  L1_LP2_filter [10.5:1] : ZeroPole  Zeros=-2*pi*[10.5]  Poles=-2*pi*[1]  Gain=[1/10.5]
  L1_LP3_filter [10.5:1] : ZeroPole  Zeros=-2*pi*[10.5]  Poles=-2*pi*[1]  Gain=[1/10.5]
  L1_Output_filter [50:300] : ZeroPole  Zeros=-2*pi*[50]  Poles=-2*pi*[300]  Gain=[300/50]
  Switch : Switch  Threshold=0.5
  Switch1 : Switch  Threshold=0.5
  Switch2 : Switch  Threshold=0.5
  drivers.uim.state.lp1 : Constant  Value=ifoParams.act.drivers.uim.state.lp1
  drivers.uim.state.lp2 : Constant  Value=ifoParams.act.drivers.uim.state.lp2
  drivers.uim.state.lp3 : Constant  Value=ifoParams.act.drivers.uim.state.lp3
  Out [A] : Outport
  wires:
  DC Transconductance/1 -> L1_LP1_filter [10.5:1]/1, Switch/3
  drivers.uim.state.lp1/1 -> Switch/2
  L1_LP1_filter [10.5:1]/1 -> Switch/1
  Switch/1 -> L1_LP2_filter [10.5:1]/1, Switch1/3
  L1_LP2_filter [10.5:1]/1 -> Switch1/1
  drivers.uim.state.lp2/1 -> Switch1/2
  Switch1/1 -> L1_LP3_filter [10.5:1]/1, Switch2/3
  L1_LP3_filter [10.5:1]/1 -> Switch2/1
  drivers.uim.state.lp3/1 -> Switch2/2
  In [V]/1 -> DC Transconductance/1
  Switch2/1 -> L1_Output_filter [50:300]/1
  L1_Output_filter [50:300]/1 -> Out [A]/1

== system DARM/Actuation Function/ETMY/Hierarchy Loops/COILOUTF/L1 ==
  note: Switches pass upper path if set to 1 (one),
      | lower path if set to 0 (zero)
  In [ct] : Inport
  Switch : Switch  Threshold=0.5
  Switch1 : Switch  Threshold=0.5
  Switch2 : Switch  Threshold=0.5
  antiAcq [10:1] : ZeroPole  Zeros=-2*pi*[300]  Poles=-2*pi*[50]  Gain=[50/300]
  antiLP1 [1:10.5] : ZeroPole  Zeros=-2*pi*[1]  Poles=-2*pi*[10.5]  Gain=[10.5/1]
  antiLP2 [1:10.5] : ZeroPole  Zeros=-2*pi*[1]  Poles=-2*pi*[10.5]  Gain=[10.5/1]
  antiLP3 [1:10.5] : ZeroPole  Zeros=-2*pi*[1]  Poles=-2*pi*[10.5]  Gain=[10.5/1]
  drivers.uim.state.lp1 : Constant  Value=ifoParams.act.drivers.uim.state.lp1
  drivers.uim.state.lp2 : Constant  Value=ifoParams.act.drivers.uim.state.lp2
  drivers.uim.state.lp3 : Constant  Value=ifoParams.act.drivers.uim.state.lp3
  Out [ct] : Outport
  wires:
  drivers.uim.state.lp1/1 -> Switch/2
  antiLP1 [1:10.5]/1 -> Switch/1
  Switch/1 -> Switch1/3, antiLP2 [1:10.5]/1
  antiLP2 [1:10.5]/1 -> Switch1/1
  drivers.uim.state.lp2/1 -> Switch1/2
  Switch1/1 -> Switch2/3, antiLP3 [1:10.5]/1
  antiLP3 [1:10.5]/1 -> Switch2/1
  drivers.uim.state.lp3/1 -> Switch2/2
  In [ct]/1 -> antiLP1 [1:10.5]/1, Switch/3
  Switch2/1 -> antiAcq [10:1]/1
  antiAcq [10:1]/1 -> Out [ct]/1

== system DARM/Actuation Function/ETMY/Hierarchy Loops/COILOUTF/L2 ==
  note: Switches pass upper path if set to 1 (one),
      | lower path if set to 0 (zero)
  In [ct] : Inport
  Switch : Switch  Threshold=0.5
  Switch1 : Switch  Threshold=0.5
  antiAcqOff [110:12] : ZeroPole  Zeros=-2*pi*[110]  Poles=-2*pi*[12]  Gain=12/110
  antiAcqOn [80.5:1.35] : ZeroPole  Zeros=-2*pi*[80.5]  Poles=-2*pi*[1.35]  Gain=1.35/80.5
  antiLpOn [(0.5 250):(6 20)] : ZeroPole  Zeros=-2*pi*[0.5 250]  Poles=-2*pi*[6 20]  Gain=(6*20)/(0.5*250)
  drivers.pum.state.lp : Constant  Value=ifoParams.act.drivers.pum.state.lp
  drivers.top.state.acq : Constant  Value=ifoParams.act.drivers.pum.state.acq
  Out [ct] : Outport
  wires:
  drivers.pum.state.lp/1 -> Switch/2
  Switch/1 -> antiAcqOn [80.5:1.35]/1, antiAcqOff [110:12]/1
  antiAcqOn [80.5:1.35]/1 -> Switch1/1
  drivers.top.state.acq/1 -> Switch1/2
  In [ct]/1 -> antiLpOn [(0.5 250):(6 20)]/1, Switch/3
  Switch1/1 -> Out [ct]/1
  antiLpOn [(0.5 250):(6 20)]/1 -> Switch/1
  antiAcqOff [110:12]/1 -> Switch1/3

== system DARM/Actuation Function/ETMY/Hierarchy Loops/COILOUTF/L3 ==
  note: 2 kHz Pole is not digitally compensated
  Ctrl In [V] : Inport
  Bias In [V] : Inport  Port=2
  Ctrl Out [V] : Outport
  Bias Out [V] : Outport  Port=2
  wires:
  Ctrl In [V]/1 -> Ctrl Out [V]/1
  Bias In [V]/1 -> Bias Out [V]/1

== system DARM/Actuation Function/ETMY/Hierarchy Loops/COILOUTF/M0 ==
  note: Switches pass upper path if set to 1 (one),
      | lower path if set to 0 (zero)
  In [ct] : Inport
  Switch : Switch  Threshold=0.5
  antiAcq [1:31] : ZeroPole  Zeros=-2*pi*[1]  Poles=-2*pi*[31]  Gain=[31/1]
  antiLP [1:10] : ZeroPole  Zeros=-2*pi*[1]  Poles=-2*pi*[10]  Gain=[10/1]
  drivers.top.state.lp : Constant  Value=ifoParams.act.drivers.top.state.lp
  Out [ct] : Outport
  wires:
  Switch/1 -> antiAcq [1:31]/1
  antiLP [1:10]/1 -> Switch/1
  In [ct]/1 -> antiLP [1:10]/1, Switch/3
  antiAcq [1:31]/1 -> Out [ct]/1
  drivers.top.state.lp/1 -> Switch/2

== system DARM/Actuation Function/ETMY/Hierarchy Loops/Driver Electronics/ESD Driver ==
  Ctrl In [V] : Inport
  Bias In [V] : Inport  Port=2
  DC Gain1 : Gain  Gain=1.1
  DC Gain3 : Gain  Gain=1.1
  L3_ESD_filter [(none):(2000)] : ZeroPole  Zeros=[]  Poles=-2*pi*[2000]  Gain=[2*pi*2000]
  L3_ESD_filter [(none):(2000)]1 : ZeroPole  Zeros=[]  Poles=-2*pi*[2000]  Gain=[2*pi*2000]
  Ctrl Out [V] : Outport
  Bias Out [V] : Outport  Port=2
  wires:
  DC Gain3/1 -> L3_ESD_filter [(none):(2000)]/1
  Ctrl In [V]/1 -> DC Gain3/1
  L3_ESD_filter [(none):(2000)]/1 -> Ctrl Out [V]/1
  Bias In [V]/1 -> DC Gain1/1
  DC Gain1/1 -> L3_ESD_filter [(none):(2000)]1/1
  L3_ESD_filter [(none):(2000)]1/1 -> Bias Out [V]/1

== system DARM/Actuation Function/ETMY/Hierarchy Loops/Driver Electronics/PUM Driver ==
  note: Switches pass upper path if set to 1 (one),
      | lower path if set to 0 (zero)
  In [V] : Inport
  DC Transconductance : Gain  Gain=0.27e-3
  L2_ACQOFF_filter [12:110] : ZeroPole  Zeros=-2*pi*[12]  Poles=-2*pi*[110]  Gain=110/12
  L2_ACQON_filter [1.35:80.5] : ZeroPole  Zeros=-2*pi*[1.35]  Poles=-2*pi*[80.5]  Gain=80.5/1.35
  L2_LPON_filter [(0.5 250):(6 20)] : ZeroPole  Zeros=-2*pi*[6 20]  Poles=-2*pi*[0.5 250]  Gain=(0.5*250)/(6*20)
  Switch : Switch  Threshold=0.5
  Switch1 : Switch  Threshold=0.5
  drivers.pum.state.lp : Constant  Value=ifoParams.act.drivers.pum.state.lp
  drivers.top.state.acq : Constant  Value=ifoParams.act.drivers.pum.state.acq
  Out [A] : Outport
  wires:
  DC Transconductance/1 -> L2_LPON_filter [(0.5 250):(6 20)]/1, Switch/3
  drivers.pum.state.lp/1 -> Switch/2
  Switch/1 -> L2_ACQOFF_filter [12:110]/1, L2_ACQON_filter [1.35:80.5]/1
  L2_ACQON_filter [1.35:80.5]/1 -> Switch1/1
  drivers.top.state.acq/1 -> Switch1/2
  In [V]/1 -> DC Transconductance/1
  Switch1/1 -> Out [A]/1
  L2_LPON_filter [(0.5 250):(6 20)]/1 -> Switch/1
  L2_ACQOFF_filter [12:110]/1 -> Switch1/3

== system DARM/Actuation Function/ETMY/Hierarchy Loops/Driver Electronics/QTOP Driver ==
  note: Switches pass upper path if set to 1 (one),
      | lower path if set to 0 (zero)
  In [V] : Inport
  DC Transconductance : Gain  Gain=9.9e-3
  LP_filter [10:1] : ZeroPole  Zeros=-2*pi*[10]  Poles=-2*pi*[1]  Gain=[1/10]
  M0_Output_Filter [31:0.9] : ZeroPole  Zeros=-2*pi*[31]  Poles=-2*pi*[0.9]  Gain=[0.9/31]
  Switch : Switch  Threshold=0.5
  drivers.top.state.lp : Constant  Value=ifoParams.act.drivers.top.state.lp
  Out [A] : Outport
  wires:
  Switch/1 -> M0_Output_Filter [31:0.9]/1
  LP_filter [10:1]/1 -> Switch/1
  DC Transconductance/1 -> LP_filter [10:1]/1, Switch/3
  In [V]/1 -> DC Transconductance/1
  M0_Output_Filter [31:0.9]/1 -> Out [A]/1
  drivers.top.state.lp/1 -> Switch/2

== system DARM/Actuation Function/ETMY/Hierarchy Loops/Driver Electronics/UIM Driver ==
  note: Switches pass upper path if set to 1 (one),
      | lower path if set to 0 (zero)
  In [V] : Inport
  DC Transconductance : Gain  Gain=0.15e-3
  L1_LP1_filter [10.5:1] : ZeroPole  Zeros=-2*pi*[10.5]  Poles=-2*pi*[1]  Gain=[1/10.5]
  L1_LP2_filter [10.5:1] : ZeroPole  Zeros=-2*pi*[10.5]  Poles=-2*pi*[1]  Gain=[1/10.5]
  L1_LP3_filter [10.5:1] : ZeroPole  Zeros=-2*pi*[10.5]  Poles=-2*pi*[1]  Gain=[1/10.5]
  L1_Output_filter [50:300] : ZeroPole  Zeros=-2*pi*[50]  Poles=-2*pi*[300]  Gain=[300/50]
  Switch : Switch  Threshold=0.5
  Switch1 : Switch  Threshold=0.5
  Switch2 : Switch  Threshold=0.5
  drivers.uim.state.lp1 : Constant  Value=ifoParams.act.drivers.uim.state.lp1
  drivers.uim.state.lp2 : Constant  Value=ifoParams.act.drivers.uim.state.lp2
  drivers.uim.state.lp3 : Constant  Value=ifoParams.act.drivers.uim.state.lp3
  Out [A] : Outport
  wires:
  DC Transconductance/1 -> L1_LP1_filter [10.5:1]/1, Switch/3
  drivers.uim.state.lp1/1 -> Switch/2
  L1_LP1_filter [10.5:1]/1 -> Switch/1
  Switch/1 -> L1_LP2_filter [10.5:1]/1, Switch1/3
  L1_LP2_filter [10.5:1]/1 -> Switch1/1
  drivers.uim.state.lp2/1 -> Switch1/2
  Switch1/1 -> L1_LP3_filter [10.5:1]/1, Switch2/3
  L1_LP3_filter [10.5:1]/1 -> Switch2/1
  drivers.uim.state.lp3/1 -> Switch2/2
  In [V]/1 -> DC Transconductance/1
  Switch2/1 -> L1_Output_filter [50:300]/1
  L1_Output_filter [50:300]/1 -> Out [A]/1
